simulink model "ProgettoLQR"  (R2021a)
settings: Solver=VariableStepAuto  StartTime=0.0  StopTime=30  RelTol=1e-3
undefined symbols (not defined in the file): A, B, K, Kinf
settings Model: Creator=a15le  LastModifiedBy=a15le

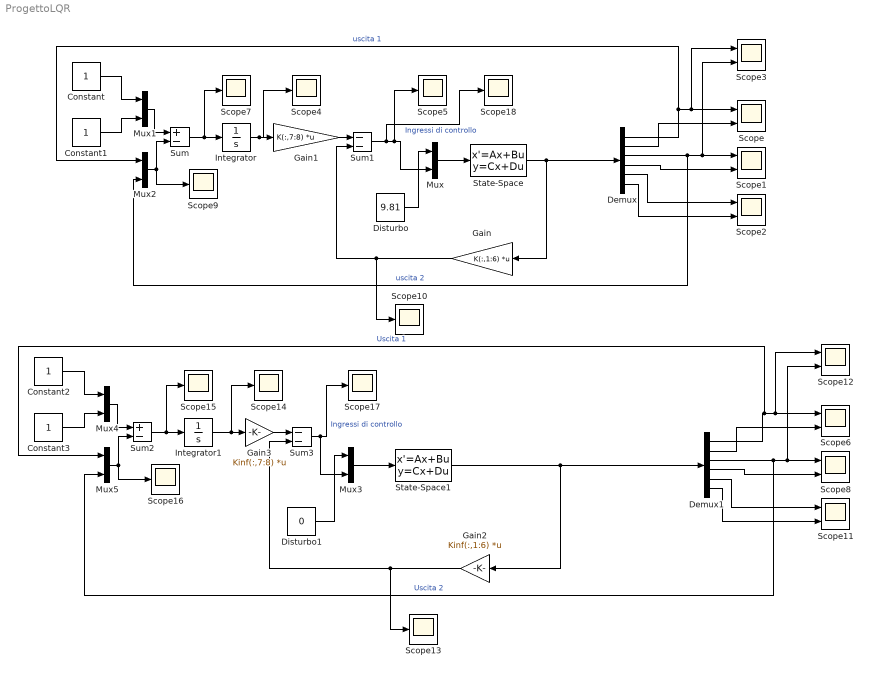
== system ProgettoLQR ==
  Constant{,1..3} (4 alike) : Constant
  Demux : Demux  Outputs=[1 1 1 1 1 1]
  Demux1 : Demux  Outputs=[1 1 1 1 1 1]
  Disturbo : Constant  Value=9.81
  Disturbo1 : Constant  Value=0
  Gain : Gain  Gain=K(:,1:6)  Multiplication=Matrix(K*u)
  Gain1 : Gain  Gain=K(:,7:8)  Multiplication=Matrix(K*u)
  Gain2 : Gain  Gain=Kinf(:,1:6)  Multiplication=Matrix(K*u)
  Gain3 : Gain  Gain=Kinf(:,7:8)  Multiplication=Matrix(K*u)
  Integrator : Integrator
  Integrator1 : Integrator
  Mux{,1..5} (6 alike) : Mux  Inputs=2
  Scope{,1..3,6,8,11..12} (8 alike) : Scope  NumInputPorts=2
  Scope{4..5,7,9..10,13..18} (11 alike) : Scope
  State-Space : StateSpace  A=A  B=B  C=eye(6)  D=zeros(6,3)  InitialCondition=[0.5;0;0.5;0;0.5;0]*0
  State-Space1 : StateSpace  A=A  B=B  C=eye(6)  D=zeros(6,3)  InitialCondition=[0.5;0;0.5;0;0.5;0]*0
  Sum : Sum  Inputs=+-
  Sum1 : Sum  Inputs=--
  Sum2 : Sum  Inputs=+-
  Sum3 : Sum  Inputs=--
  wires:
  State-Space/1 -> Gain/1, Demux/1
  Mux/1 -> State-Space/1
  Sum/1 -> Scope7/1, Integrator/1
  Integrator/1 -> Scope4/1, Gain1/1
  Gain1/1 -> Sum1/1
  Sum1/1 -> Scope18/1, Mux/2, Scope5/1  "Ingressi di controllo"
  Disturbo/1 -> Mux/1
  Gain/1 -> Scope10/1, Sum1/2
  Constant/1 -> Mux1/1
  Constant1/1 -> Mux1/2
  Demux/1 -> Mux2/1, Scope3/1, Scope/1  "uscita 1"
  Demux/2 -> Scope/2
  Demux/3 -> Mux2/2, Scope3/2, Scope1/1  "uscita 2"
  Demux/4 -> Scope1/2
  Demux/6 -> Scope2/2
  Mux2/1 -> Sum/2, Scope9/1
  Demux/5 -> Scope2/1
  Mux1/1 -> Sum/1
  Demux1/6 -> Scope11/2
  Demux1/2 -> Scope6/2
  Demux1/5 -> Scope11/1
  Demux1/4 -> Scope8/2
  State-Space1/1 -> Gain2/1, Demux1/1
  Gain2/1 -> Scope13/1, Sum3/2
  Mux3/1 -> State-Space1/1
  Disturbo1/1 -> Mux3/1
  Sum2/1 -> Scope15/1, Integrator1/1
  Integrator1/1 -> Scope14/1, Gain3/1
  Gain3/1 -> Sum3/1
  Mux5/1 -> Scope16/1, Sum2/2
  Demux1/3 -> Mux5/2, Scope12/2, Scope8/1  "Uscita 2"
  Mux4/1 -> Sum2/1
  Constant3/1 -> Mux4/2
  Demux1/1 -> Mux5/1, Scope12/1, Scope6/1  "Uscita 1"
  Constant2/1 -> Mux4/1
  Sum3/1 -> Scope17/1, Mux3/2  "Ingressi di controllo"
